simulink model "llr"  (R2020b)
settings: Solver=VariableStepAuto  StartTime=0.0  StopTime=20  RelTol=1e-3
values from neighbouring files (symbols this model uses):
  fs = 160e6    (= 160000000)    [setup.m]
libraries: simulink x14, hdlsllib x6, dspsigops x4, dspsrcs4 x3
settings Model: Creator=ckb13136  LastModifiedBy=ckb13136

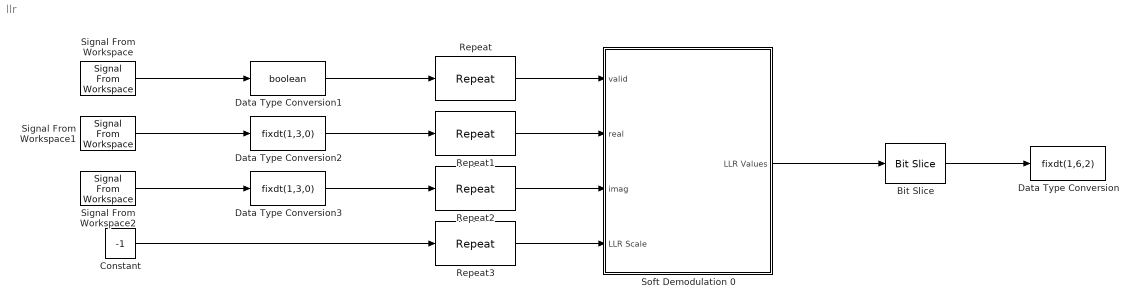
== system llr ==
  Bit Slice : hdlsllib/Logic and Bit Operations/Bit Slice  lidx=5  ridx=0
      settings: SourceProductBaseCode=SL
  Constant : Constant  Value=-1  OutDataTypeStr=fixdt(1,32,22)  SampleTime=1
  Data Type Conversion : DataTypeConversion  OutDataTypeStr=fixdt(1,6,2)  ConvertRealWorld=Stored Integer (SI)
  Data Type Conversion1 : DataTypeConversion  OutDataTypeStr=boolean
  Data Type Conversion2 : DataTypeConversion  OutDataTypeStr=fixdt(1,3,0)
  Data Type Conversion3 : DataTypeConversion  OutDataTypeStr=fixdt(1,3,0)
  Repeat{,1..3} (4 alike) : dspsigops/Repeat  N=4  InputProcessing=Columns as channels (frame based)  RateOptions=Allow multirate processing  ic=0  mode=Unused parameter value
      settings: SourceProductName=DSP System Toolbox
  Signal From Workspace : dspsrcs4/Signal From Workspace  X=ones(1,16)  Ts=1  nsamps=1  OutputAfterFinalValue=Setting to zero  ignoreOrWarnInputAndFrameLengths=off  OutputFrames=off
  Signal From Workspace1 : dspsrcs4/Signal From Workspace  X=[3 1 -1 -3 3 1 -1 -3 3 1 -1 -3 3 1 -1 -3 3 1 -1 -3 3 1 -1 -3]  Ts=1  nsamps=1  OutputAfterFinalValue=Setting to zero  ignoreOrWarnInputAndFrameLengths=off  OutputFrames=off
  Signal From Workspace2 : dspsrcs4/Signal From Workspace  X=[1 1 1 1 3 3 3 3 -1 -1 -1 -1 -3 -3 -3 -3]  Ts=1  nsamps=1  OutputAfterFinalValue=Setting to zero  ignoreOrWarnInputAndFrameLengths=off  OutputFrames=off
  Soft Demodulation 0 : Subsystem  mask{w=3, f=0, n=1}
  wires:
  Constant/1 -> Repeat3/1
  Signal From Workspace2/1 -> Data Type Conversion3/1
  Signal From Workspace1/1 -> Data Type Conversion2/1
  Signal From Workspace/1 -> Data Type Conversion1/1
  Soft Demodulation 0/1(LLR Values) -> Bit Slice/1
  Bit Slice/1 -> Data Type Conversion/1
  Repeat/1 -> Soft Demodulation 0/1(valid)
  Repeat1/1 -> Soft Demodulation 0/2(real)
  Repeat2/1 -> Soft Demodulation 0/3(imag)
  Repeat3/1 -> Soft Demodulation 0/4(LLR Scale)
  Data Type Conversion1/1 -> Repeat/1
  Data Type Conversion2/1 -> Repeat1/1
  Data Type Conversion3/1 -> Repeat2/1

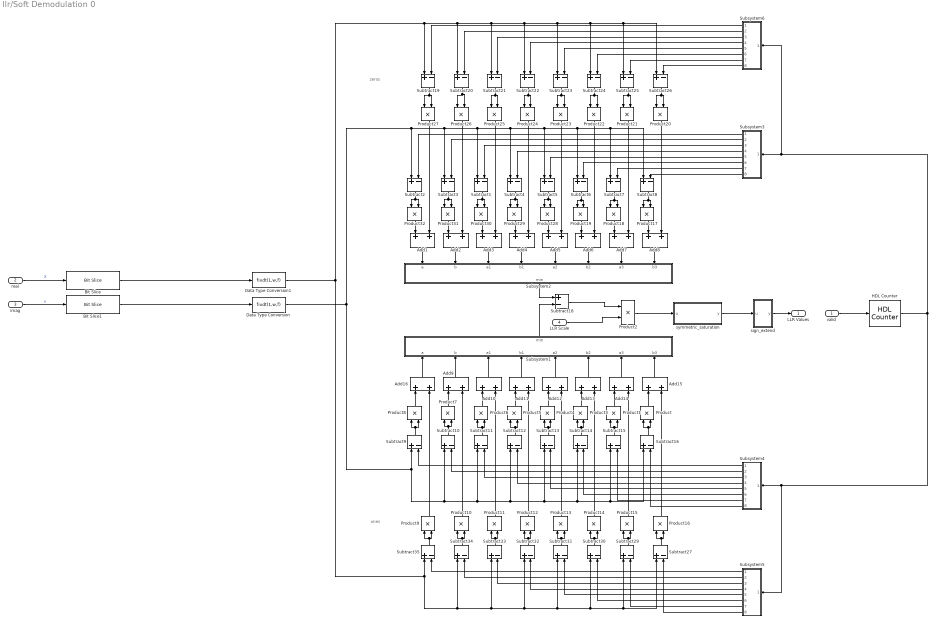
== system llr/Soft Demodulation 0 ==
  note: zeros
  note: ones
  valid : Inport
  real : Inport  Port=2
  imag : Inport  Port=3
  LLR Scale : Inport  Port=4
  Add{1..16} (16 alike) : Sum  OutDataTypeStr=fixdt(1,(w+1)*2+1,f*2)  SaturateOnIntegerOverflow=on
  Bit Slice : hdlsllib/Logic and Bit Operations/Bit Slice  lidx=(n*w)-1  ridx=(n-1)*w
      settings: SourceProductBaseCode=SL
  Bit Slice1 : hdlsllib/Logic and Bit Operations/Bit Slice  lidx=(n*w)-1  ridx=(n-1)*w
      settings: SourceProductBaseCode=SL
  Data Type Conversion : DataTypeConversion  OutDataTypeStr=fixdt(1,w,f)  ConvertRealWorld=Stored Integer (SI)
  Data Type Conversion1 : DataTypeConversion  OutDataTypeStr=fixdt(1,w,f)  ConvertRealWorld=Stored Integer (SI)
  HDL Counter : hdlsllib/Sources/HDL Counter  CountType=Count limited  CountInit=0  CountStep=1  CountMax=3  CountFromType=Initial value  CountFrom=0  CountResetPort=off  CountLoadPort=off  CountEnbPort=on  CountDirPort=off  CountDataType=Unsigned  CountWordLen=2  CountFracLen=0  CountSampTime=1/(fs*2)
  Product{,1,3..16} (16 alike) : Product  SaturateOnIntegerOverflow=on
  Product{17..32} (16 alike) : Product
  Product2 : Product  RndMeth=Round  SaturateOnIntegerOverflow=on
  Subsystem1 : Subsystem
  Subsystem2 : Subsystem
  Subsystem3 : Subsystem
  Subsystem4 : Subsystem
  Subsystem5 : Subsystem
  Subsystem6 : Subsystem
  Subtract{1..16,19..27,29..35} (32 alike) : Sum  Inputs=+-  OutDataTypeStr=fixdt(1,w+1,f)  SaturateOnIntegerOverflow=on
  Subtract18 : Sum  Inputs=+-  OutDataTypeStr=fixdt(1,(w+1)*2+2,f*2)  SaturateOnIntegerOverflow=on
  sign_extend : Subsystem
  symmetric_saturation : MATLAB Function  TreatAsAtomicUnit=on
  LLR Values : Outport
  wires:
  Subsystem5/4(Out4) -> Subtract32/2
  Product6/1 -> Add10/1
  Product10/1 -> Add9/2
  Add12/1 -> Subsystem1/5(a2)
  Product1/1 -> Add14/1
  Subtract13/1 -> Product4/1, Product4/2
  Product/1 -> Add15/1
  Add1/1 -> Subsystem2/1(a)
  Product20/1 -> Add8/2
  Add3/1 -> Subsystem2/3(a1)
  Subsystem2/1(min) -> Subtract18/1
  Subsystem3/6(Out6) -> Subtract6/2
  Subtract10/1 -> Product7/2, Product7/1
  Subtract35/1 -> Product9/2, Product9/1
  real/1 -> Bit Slice/1  "X"
  Product25/1 -> Add3/2
  Product19/1 -> Add6/1
  Product3/1 -> Add13/1
  Add7/1 -> Subsystem2/7(a3)
  Product23/1 -> Add5/2
  Subtract21/1 -> Product25/1, Product25/2
  Product4/1 -> Add12/1
  LLR Scale/1 -> Product2/2
  Add10/1 -> Subsystem1/3(a1)
  Subtract24/1 -> Product22/1, Product22/2
  Subtract1/1 -> Product30/1, Product30/2
  Subsystem4/6(Out6) -> Subtract14/2
  Subtract18/1 -> Product2/1
  Product5/1 -> Add11/1
  Subsystem1/1(min) -> Subtract18/2
  Product22/1 -> Add6/2
  Subsystem3/2(Out2) -> Subtract3/2
  Add13/1 -> Subsystem1/6(b2)
  Product26/1 -> Add2/2
  Subtract19/1 -> Product27/1, Product27/2
  Product31/1 -> Add2/1
  Subsystem3/5(Out5) -> Subtract5/2
  Product30/1 -> Add3/1
  Add15/1 -> Subsystem1/8(b3)
  Product18/1 -> Add7/1
  Subtract4/1 -> Product29/2, Product29/1
  Subtract5/1 -> Product28/1, Product28/2
  Subtract2/1 -> Product32/1, Product32/2
  Add16/1 -> Subsystem1/1(a)
  imag/1 -> Bit Slice1/1  "y"
  Add14/1 -> Subsystem1/7(a3)
  Subtract23/1 -> Product23/2, Product23/1
  Subtract15/1 -> Product1/2, Product1/1
  Subtract9/1 -> Product8/2, Product8/1
  Subsystem3/1(Out1) -> Subtract2/2
  Product27/1 -> Add1/2
  Add8/1 -> Subsystem2/8(b3)
  Product14/1 -> Add13/2
  Product15/1 -> Add14/2
  Add2/1 -> Subsystem2/2(b)
  Add11/1 -> Subsystem1/4(b1)
  Add6/1 -> Subsystem2/6(b2)
  Subtract25/1 -> Product21/1, Product21/2
  Product21/1 -> Add7/2
  Subsystem3/4(Out4) -> Subtract4/2
  Subsystem4/5(Out5) -> Subtract13/2
  Product7/1 -> Add9/1
  Product8/1 -> Add16/1
  Product12/1 -> Add11/2
  Product28/1 -> Add5/1
  Subsystem3/3(Out3) -> Subtract1/2
  Subtract26/1 -> Product20/1, Product20/2
  Subsystem4/7(Out7) -> Subtract15/2
  Add9/1 -> Subsystem1/2(b)
  Product9/1 -> Add16/2
  Subsystem4/4(Out4) -> Subtract12/2
  Product17/1 -> Add8/1
  Subsystem4/3(Out3) -> Subtract11/2
  Subsystem5/2(Out2) -> Subtract34/2
  Subsystem5/3(Out3) -> Subtract33/2
  Product13/1 -> Add12/2
  Subtract3/1 -> Product31/1, Product31/2
  Product24/1 -> Add4/2
  Subsystem5/6(Out6) -> Subtract30/2
  Subsystem4/1(Out1) -> Subtract9/2
  Product16/1 -> Add15/2
  Subsystem3/7(Out7) -> Subtract7/2
  Subtract12/1 -> Product5/2, Product5/1
  Subsystem5/1(Out1) -> Subtract35/2
  Product32/1 -> Add1/1
  Subtract34/1 -> Product10/2, Product10/1
  Subtract11/1 -> Product6/2, Product6/1
  Subsystem5/7(Out7) -> Subtract29/2
  Subsystem5/8(Out8) -> Subtract27/2
  Subsystem4/2(Out2) -> Subtract10/2
  Subsystem4/8(Out8) -> Subtract16/2
  Product29/1 -> Add4/1
  Product11/1 -> Add10/2
  Add4/1 -> Subsystem2/4(b1)
  Subsystem3/8(Out8) -> Subtract8/2
  Add5/1 -> Subsystem2/5(a2)
  Subtract16/1 -> Product/2, Product/1
  Subsystem5/5(Out5) -> Subtract31/2
  Subtract14/1 -> Product3/1, Product3/2
  Subtract33/1 -> Product11/1, Product11/2
  Subtract32/1 -> Product12/1, Product12/2
  Subtract31/1 -> Product13/1, Product13/2
  Subtract30/1 -> Product14/1, Product14/2
  Subtract29/1 -> Product15/1, Product15/2
  Subtract27/1 -> Product16/1, Product16/2
  Subtract8/1 -> Product17/2, Product17/1
  Subtract7/1 -> Product18/1, Product18/2
  Subtract20/1 -> Product26/2, Product26/1
  Subtract22/1 -> Product24/1, Product24/2
  Subtract6/1 -> Product19/1, Product19/2
  Subsystem6/1(Out1) -> Subtract19/2
  Subsystem6/2(Out2) -> Subtract20/2
  Subsystem6/3(Out3) -> Subtract21/2
  Subsystem6/4(Out4) -> Subtract22/2
  Subsystem6/5(Out5) -> Subtract23/2
  Subsystem6/6(Out6) -> Subtract24/2
  Subsystem6/7(Out7) -> Subtract25/2
  Subsystem6/8(Out8) -> Subtract26/2
  valid/1 -> HDL Counter/1
  HDL Counter/1 -> Subsystem5/1(enb), Subsystem4/1(enb), Subsystem6/1(enb), Subsystem3/1(enb)
  symmetric_saturation/1(y) -> sign_extend/1(u)
  Product2/1 -> symmetric_saturation/1(u)
  sign_extend/1(y) -> LLR Values/1
  Data Type Conversion/1 -> Subtract2/1, Subtract3/1, Subtract1/1, Subtract4/1, Subtract5/1, Subtract6/1, Subtract8/1, Subtract7/1, Subtract9/1, Subtract10/1, Subtract11/1, Subtract12/1, Subtract13/1, Subtract14/1, Subtract16/1, Subtract15/1
  Data Type Conversion1/1 -> Subtract19/1, Subtract21/1, Subtract22/1, Subtract23/1, Subtract24/1, Subtract25/1, Subtract26/1, Subtract20/1, Subtract35/1, Subtract34/1, Subtract33/1, Subtract32/1, Subtract31/1, Subtract30/1, Subtract29/1, Subtract27/1
  Bit Slice1/1 -> Data Type Conversion/1
  Bit Slice/1 -> Data Type Conversion1/1

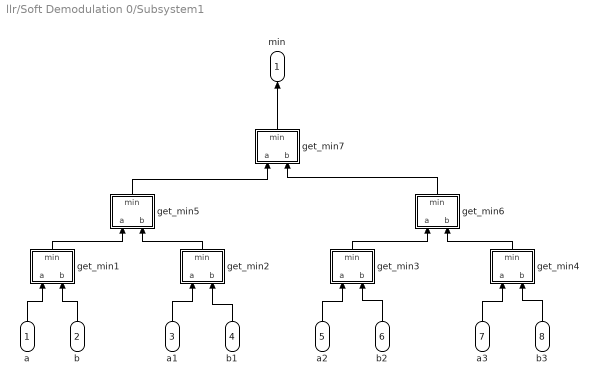
== system llr/Soft Demodulation 0/Subsystem1 ==
  a : Inport
  b : Inport  Port=2
  a1 : Inport  Port=3
  b1 : Inport  Port=4
  a2 : Inport  Port=5
  b2 : Inport  Port=6
  a3 : Inport  Port=7
  b3 : Inport  Port=8
  get_min1 : Subsystem
  get_min2 : Subsystem
  get_min3 : Subsystem
  get_min4 : Subsystem
  get_min5 : Subsystem
  get_min6 : Subsystem
  get_min7 : Subsystem
  min : Outport
  wires:
  get_min5/1(min) -> get_min7/1(a)
  b2/1 -> get_min3/2(b)
  a/1 -> get_min1/1(a)
  get_min6/1(min) -> get_min7/2(b)
  get_min3/1(min) -> get_min6/1(a)
  b1/1 -> get_min2/2(b)
  get_min2/1(min) -> get_min5/2(b)
  get_min4/1(min) -> get_min6/2(b)
  a3/1 -> get_min4/1(a)
  get_min1/1(min) -> get_min5/1(a)
  get_min7/1(min) -> min/1
  b3/1 -> get_min4/2(b)
  a1/1 -> get_min2/1(a)
  b/1 -> get_min1/2(b)
  a2/1 -> get_min3/1(a)

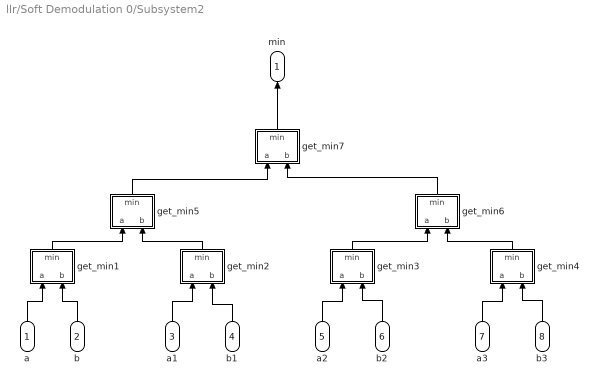
== system llr/Soft Demodulation 0/Subsystem2 ==
  a : Inport
  b : Inport  Port=2
  a1 : Inport  Port=3
  b1 : Inport  Port=4
  a2 : Inport  Port=5
  b2 : Inport  Port=6
  a3 : Inport  Port=7
  b3 : Inport  Port=8
  get_min1 : Subsystem
  get_min2 : Subsystem
  get_min3 : Subsystem
  get_min4 : Subsystem
  get_min5 : Subsystem
  get_min6 : Subsystem
  get_min7 : Subsystem
  min : Outport
  wires:
  get_min5/1(min) -> get_min7/1(a)
  b2/1 -> get_min3/2(b)
  a/1 -> get_min1/1(a)
  get_min6/1(min) -> get_min7/2(b)
  get_min3/1(min) -> get_min6/1(a)
  b1/1 -> get_min2/2(b)
  get_min2/1(min) -> get_min5/2(b)
  get_min4/1(min) -> get_min6/2(b)
  a3/1 -> get_min4/1(a)
  get_min1/1(min) -> get_min5/1(a)
  get_min7/1(min) -> min/1
  b3/1 -> get_min4/2(b)
  a1/1 -> get_min2/1(a)
  b/1 -> get_min1/2(b)
  a2/1 -> get_min3/1(a)

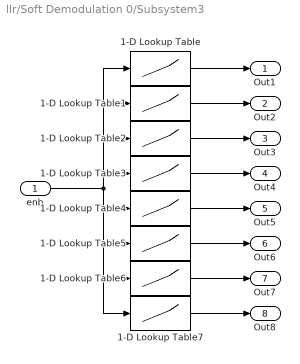
== system llr/Soft Demodulation 0/Subsystem3 ==
  enb : Inport
  1-D Lookup Table : Lookup_n-D  NumberOfTableDimensions=1  BreakpointsForDimension1=[0:3]  IndexSearchMethod=Evenly spaced points  Table=z_y(1:8:end)  InterpMethod=Flat  DiagnosticForOutOfRangeInput=Error  InternalRulePriority=Speed  OutDataTypeStr=fixdt(1,3,0)  RndMeth=Simplest  InputSameDT=on
  1-D Lookup Table1 : Lookup_n-D  NumberOfTableDimensions=1  BreakpointsForDimension1=[0:3]  IndexSearchMethod=Evenly spaced points  Table=z_y(2:8:end)  InterpMethod=Flat  DiagnosticForOutOfRangeInput=Error  InternalRulePriority=Speed  OutDataTypeStr=fixdt(1,3,0)  RndMeth=Simplest  InputSameDT=on
  1-D Lookup Table2 : Lookup_n-D  NumberOfTableDimensions=1  BreakpointsForDimension1=[0:3]  IndexSearchMethod=Evenly spaced points  Table=z_y(3:8:end)  InterpMethod=Flat  DiagnosticForOutOfRangeInput=Error  InternalRulePriority=Speed  OutDataTypeStr=fixdt(1,3,0)  RndMeth=Simplest  InputSameDT=on
  1-D Lookup Table3 : Lookup_n-D  NumberOfTableDimensions=1  BreakpointsForDimension1=[0:3]  IndexSearchMethod=Evenly spaced points  Table=z_y(4:8:end)  InterpMethod=Flat  DiagnosticForOutOfRangeInput=Error  InternalRulePriority=Speed  OutDataTypeStr=fixdt(1,3,0)  RndMeth=Simplest  InputSameDT=on
  1-D Lookup Table4 : Lookup_n-D  NumberOfTableDimensions=1  BreakpointsForDimension1=[0:3]  IndexSearchMethod=Evenly spaced points  Table=z_y(5:8:end)  InterpMethod=Flat  DiagnosticForOutOfRangeInput=Error  InternalRulePriority=Speed  OutDataTypeStr=fixdt(1,3,0)  RndMeth=Simplest  InputSameDT=on
  1-D Lookup Table5 : Lookup_n-D  NumberOfTableDimensions=1  BreakpointsForDimension1=[0:3]  IndexSearchMethod=Evenly spaced points  Table=z_y(6:8:end)  InterpMethod=Flat  DiagnosticForOutOfRangeInput=Error  InternalRulePriority=Speed  OutDataTypeStr=fixdt(1,3,0)  RndMeth=Simplest  InputSameDT=on
  1-D Lookup Table6 : Lookup_n-D  NumberOfTableDimensions=1  BreakpointsForDimension1=[0:3]  IndexSearchMethod=Evenly spaced points  Table=z_y(7:8:end)  InterpMethod=Flat  DiagnosticForOutOfRangeInput=Error  InternalRulePriority=Speed  OutDataTypeStr=fixdt(1,3,0)  RndMeth=Simplest  InputSameDT=on
  1-D Lookup Table7 : Lookup_n-D  NumberOfTableDimensions=1  BreakpointsForDimension1=[0:3]  IndexSearchMethod=Evenly spaced points  Table=z_y(8:8:end)  InterpMethod=Flat  DiagnosticForOutOfRangeInput=Error  InternalRulePriority=Speed  OutDataTypeStr=fixdt(1,3,0)  RndMeth=Simplest  InputSameDT=on
  Out1 : Outport
  Out2 : Outport  Port=2
  Out3 : Outport  Port=3
  Out4 : Outport  Port=4
  Out5 : Outport  Port=5
  Out6 : Outport  Port=6
  Out7 : Outport  Port=7
  Out8 : Outport  Port=8
  wires:
  1-D Lookup Table6/1 -> Out7/1
  enb/1 -> 1-D Lookup Table4/1, 1-D Lookup Table5/1, 1-D Lookup Table6/1, 1-D Lookup Table7/1, 1-D Lookup Table/1, 1-D Lookup Table1/1, 1-D Lookup Table2/1, 1-D Lookup Table3/1
  1-D Lookup Table3/1 -> Out4/1
  1-D Lookup Table1/1 -> Out2/1
  1-D Lookup Table4/1 -> Out5/1
  1-D Lookup Table5/1 -> Out6/1
  1-D Lookup Table/1 -> Out1/1
  1-D Lookup Table2/1 -> Out3/1
  1-D Lookup Table7/1 -> Out8/1

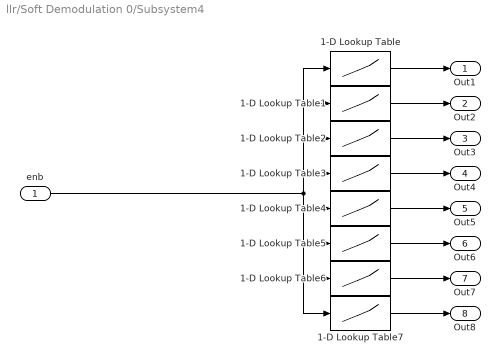
== system llr/Soft Demodulation 0/Subsystem4 ==
  enb : Inport
  1-D Lookup Table : Lookup_n-D  NumberOfTableDimensions=1  BreakpointsForDimension1=[0:3]  IndexSearchMethod=Evenly spaced points  Table=o_y(1:8:end)  InterpMethod=Flat  DiagnosticForOutOfRangeInput=Error  InternalRulePriority=Speed  OutDataTypeStr=fixdt(1,3,0)  RndMeth=Simplest  InputSameDT=on
  1-D Lookup Table1 : Lookup_n-D  NumberOfTableDimensions=1  BreakpointsForDimension1=[0:3]  IndexSearchMethod=Evenly spaced points  Table=o_y(2:8:end)  InterpMethod=Flat  DiagnosticForOutOfRangeInput=Error  InternalRulePriority=Speed  OutDataTypeStr=fixdt(1,3,0)  RndMeth=Simplest  InputSameDT=on
  1-D Lookup Table2 : Lookup_n-D  NumberOfTableDimensions=1  BreakpointsForDimension1=[0:3]  IndexSearchMethod=Evenly spaced points  Table=o_y(3:8:end)  InterpMethod=Flat  DiagnosticForOutOfRangeInput=Error  InternalRulePriority=Speed  OutDataTypeStr=fixdt(1,3,0)  RndMeth=Simplest  InputSameDT=on
  1-D Lookup Table3 : Lookup_n-D  NumberOfTableDimensions=1  BreakpointsForDimension1=[0:3]  IndexSearchMethod=Evenly spaced points  Table=o_y(4:8:end)  InterpMethod=Flat  DiagnosticForOutOfRangeInput=Error  InternalRulePriority=Speed  OutDataTypeStr=fixdt(1,3,0)  RndMeth=Simplest  InputSameDT=on
  1-D Lookup Table4 : Lookup_n-D  NumberOfTableDimensions=1  BreakpointsForDimension1=[0:3]  IndexSearchMethod=Evenly spaced points  Table=o_y(5:8:end)  InterpMethod=Flat  DiagnosticForOutOfRangeInput=Error  InternalRulePriority=Speed  OutDataTypeStr=fixdt(1,3,0)  RndMeth=Simplest  InputSameDT=on
  1-D Lookup Table5 : Lookup_n-D  NumberOfTableDimensions=1  BreakpointsForDimension1=[0:3]  IndexSearchMethod=Evenly spaced points  Table=o_y(6:8:end)  InterpMethod=Flat  DiagnosticForOutOfRangeInput=Error  InternalRulePriority=Speed  OutDataTypeStr=fixdt(1,3,0)  RndMeth=Simplest  InputSameDT=on
  1-D Lookup Table6 : Lookup_n-D  NumberOfTableDimensions=1  BreakpointsForDimension1=[0:3]  IndexSearchMethod=Evenly spaced points  Table=o_y(7:8:end)  InterpMethod=Flat  DiagnosticForOutOfRangeInput=Error  InternalRulePriority=Speed  OutDataTypeStr=fixdt(1,3,0)  RndMeth=Simplest  InputSameDT=on
  1-D Lookup Table7 : Lookup_n-D  NumberOfTableDimensions=1  BreakpointsForDimension1=[0:3]  IndexSearchMethod=Evenly spaced points  Table=o_y(8:8:end)  InterpMethod=Flat  DiagnosticForOutOfRangeInput=Error  InternalRulePriority=Speed  OutDataTypeStr=fixdt(1,3,0)  RndMeth=Simplest  InputSameDT=on
  Out1 : Outport
  Out2 : Outport  Port=2
  Out3 : Outport  Port=3
  Out4 : Outport  Port=4
  Out5 : Outport  Port=5
  Out6 : Outport  Port=6
  Out7 : Outport  Port=7
  Out8 : Outport  Port=8
  wires:
  1-D Lookup Table7/1 -> Out8/1
  1-D Lookup Table2/1 -> Out3/1
  1-D Lookup Table/1 -> Out1/1
  1-D Lookup Table5/1 -> Out6/1
  1-D Lookup Table4/1 -> Out5/1
  1-D Lookup Table1/1 -> Out2/1
  1-D Lookup Table3/1 -> Out4/1
  enb/1 -> 1-D Lookup Table7/1, 1-D Lookup Table6/1, 1-D Lookup Table5/1, 1-D Lookup Table4/1, 1-D Lookup Table3/1, 1-D Lookup Table2/1, 1-D Lookup Table1/1, 1-D Lookup Table/1
  1-D Lookup Table6/1 -> Out7/1

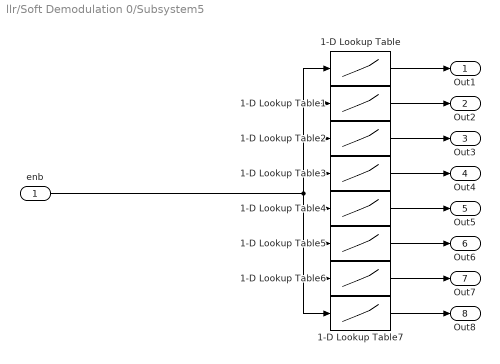
== system llr/Soft Demodulation 0/Subsystem5 ==
  enb : Inport
  1-D Lookup Table : Lookup_n-D  NumberOfTableDimensions=1  BreakpointsForDimension1=[0:3]  IndexSearchMethod=Evenly spaced points  Table=o_x(1:8:end)  InterpMethod=Flat  DiagnosticForOutOfRangeInput=Error  InternalRulePriority=Speed  OutDataTypeStr=fixdt(1,3,0)  RndMeth=Simplest  InputSameDT=on
  1-D Lookup Table1 : Lookup_n-D  NumberOfTableDimensions=1  BreakpointsForDimension1=[0:3]  IndexSearchMethod=Evenly spaced points  Table=o_x(2:8:end)  InterpMethod=Flat  DiagnosticForOutOfRangeInput=Error  InternalRulePriority=Speed  OutDataTypeStr=fixdt(1,3,0)  RndMeth=Simplest  InputSameDT=on
  1-D Lookup Table2 : Lookup_n-D  NumberOfTableDimensions=1  BreakpointsForDimension1=[0:3]  IndexSearchMethod=Evenly spaced points  Table=o_x(3:8:end)  InterpMethod=Flat  DiagnosticForOutOfRangeInput=Error  InternalRulePriority=Speed  OutDataTypeStr=fixdt(1,3,0)  RndMeth=Simplest  InputSameDT=on
  1-D Lookup Table3 : Lookup_n-D  NumberOfTableDimensions=1  BreakpointsForDimension1=[0:3]  IndexSearchMethod=Evenly spaced points  Table=o_x(4:8:end)  InterpMethod=Flat  DiagnosticForOutOfRangeInput=Error  InternalRulePriority=Speed  OutDataTypeStr=fixdt(1,3,0)  RndMeth=Simplest  InputSameDT=on
  1-D Lookup Table4 : Lookup_n-D  NumberOfTableDimensions=1  BreakpointsForDimension1=[0:3]  IndexSearchMethod=Evenly spaced points  Table=o_x(5:8:end)  InterpMethod=Flat  DiagnosticForOutOfRangeInput=Error  InternalRulePriority=Speed  OutDataTypeStr=fixdt(1,3,0)  RndMeth=Simplest  InputSameDT=on
  1-D Lookup Table5 : Lookup_n-D  NumberOfTableDimensions=1  BreakpointsForDimension1=[0:3]  IndexSearchMethod=Evenly spaced points  Table=o_x(6:8:end)  InterpMethod=Flat  DiagnosticForOutOfRangeInput=Error  InternalRulePriority=Speed  OutDataTypeStr=fixdt(1,3,0)  RndMeth=Simplest  InputSameDT=on
  1-D Lookup Table6 : Lookup_n-D  NumberOfTableDimensions=1  BreakpointsForDimension1=[0:3]  IndexSearchMethod=Evenly spaced points  Table=o_x(7:8:end)  InterpMethod=Flat  DiagnosticForOutOfRangeInput=Error  InternalRulePriority=Speed  OutDataTypeStr=fixdt(1,3,0)  RndMeth=Simplest  InputSameDT=on
  1-D Lookup Table7 : Lookup_n-D  NumberOfTableDimensions=1  BreakpointsForDimension1=[0:3]  IndexSearchMethod=Evenly spaced points  Table=o_x(8:8:end)  InterpMethod=Flat  DiagnosticForOutOfRangeInput=Error  InternalRulePriority=Speed  OutDataTypeStr=fixdt(1,3,0)  RndMeth=Simplest  InputSameDT=on
  Out1 : Outport
  Out2 : Outport  Port=2
  Out3 : Outport  Port=3
  Out4 : Outport  Port=4
  Out5 : Outport  Port=5
  Out6 : Outport  Port=6
  Out7 : Outport  Port=7
  Out8 : Outport  Port=8
  wires:
  1-D Lookup Table6/1 -> Out7/1
  enb/1 -> 1-D Lookup Table/1, 1-D Lookup Table1/1, 1-D Lookup Table2/1, 1-D Lookup Table3/1, 1-D Lookup Table4/1, 1-D Lookup Table5/1, 1-D Lookup Table6/1, 1-D Lookup Table7/1
  1-D Lookup Table3/1 -> Out4/1
  1-D Lookup Table1/1 -> Out2/1
  1-D Lookup Table4/1 -> Out5/1
  1-D Lookup Table5/1 -> Out6/1
  1-D Lookup Table/1 -> Out1/1
  1-D Lookup Table2/1 -> Out3/1
  1-D Lookup Table7/1 -> Out8/1

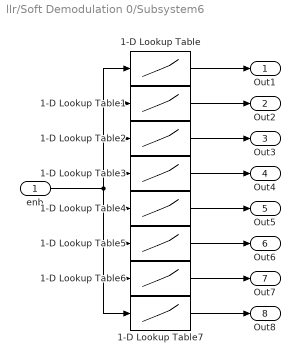
== system llr/Soft Demodulation 0/Subsystem6 ==
  enb : Inport
  1-D Lookup Table : Lookup_n-D  NumberOfTableDimensions=1  BreakpointsForDimension1=[0:3]  IndexSearchMethod=Evenly spaced points  Table=z_x(1:8:end)  InterpMethod=Flat  DiagnosticForOutOfRangeInput=Error  InternalRulePriority=Speed  OutDataTypeStr=fixdt(1,3,0)  RndMeth=Simplest  InputSameDT=on
  1-D Lookup Table1 : Lookup_n-D  NumberOfTableDimensions=1  BreakpointsForDimension1=[0:3]  IndexSearchMethod=Evenly spaced points  Table=z_x(2:8:end)  InterpMethod=Flat  DiagnosticForOutOfRangeInput=Error  InternalRulePriority=Speed  OutDataTypeStr=fixdt(1,3,0)  RndMeth=Simplest  InputSameDT=on
  1-D Lookup Table2 : Lookup_n-D  NumberOfTableDimensions=1  BreakpointsForDimension1=[0:3]  IndexSearchMethod=Evenly spaced points  Table=z_x(3:8:end)  InterpMethod=Flat  DiagnosticForOutOfRangeInput=Error  InternalRulePriority=Speed  OutDataTypeStr=fixdt(1,3,0)  RndMeth=Simplest  InputSameDT=on
  1-D Lookup Table3 : Lookup_n-D  NumberOfTableDimensions=1  BreakpointsForDimension1=[0:3]  IndexSearchMethod=Evenly spaced points  Table=z_x(4:8:end)  InterpMethod=Flat  DiagnosticForOutOfRangeInput=Error  InternalRulePriority=Speed  OutDataTypeStr=fixdt(1,3,0)  RndMeth=Simplest  InputSameDT=on
  1-D Lookup Table4 : Lookup_n-D  NumberOfTableDimensions=1  BreakpointsForDimension1=[0:3]  IndexSearchMethod=Evenly spaced points  Table=z_x(5:8:end)  InterpMethod=Flat  DiagnosticForOutOfRangeInput=Error  InternalRulePriority=Speed  OutDataTypeStr=fixdt(1,3,0)  RndMeth=Simplest  InputSameDT=on
  1-D Lookup Table5 : Lookup_n-D  NumberOfTableDimensions=1  BreakpointsForDimension1=[0:3]  IndexSearchMethod=Evenly spaced points  Table=z_x(6:8:end)  InterpMethod=Flat  DiagnosticForOutOfRangeInput=Error  InternalRulePriority=Speed  OutDataTypeStr=fixdt(1,3,0)  RndMeth=Simplest  InputSameDT=on
  1-D Lookup Table6 : Lookup_n-D  NumberOfTableDimensions=1  BreakpointsForDimension1=[0:3]  IndexSearchMethod=Evenly spaced points  Table=z_x(7:8:end)  InterpMethod=Flat  DiagnosticForOutOfRangeInput=Error  InternalRulePriority=Speed  OutDataTypeStr=fixdt(1,3,0)  RndMeth=Simplest  InputSameDT=on
  1-D Lookup Table7 : Lookup_n-D  NumberOfTableDimensions=1  BreakpointsForDimension1=[0:3]  IndexSearchMethod=Evenly spaced points  Table=z_x(8:8:end)  InterpMethod=Flat  DiagnosticForOutOfRangeInput=Error  InternalRulePriority=Speed  OutDataTypeStr=fixdt(1,3,0)  RndMeth=Simplest  InputSameDT=on
  Out1 : Outport
  Out2 : Outport  Port=2
  Out3 : Outport  Port=3
  Out4 : Outport  Port=4
  Out5 : Outport  Port=5
  Out6 : Outport  Port=6
  Out7 : Outport  Port=7
  Out8 : Outport  Port=8
  wires:
  1-D Lookup Table7/1 -> Out8/1
  1-D Lookup Table2/1 -> Out3/1
  1-D Lookup Table/1 -> Out1/1
  1-D Lookup Table5/1 -> Out6/1
  1-D Lookup Table4/1 -> Out5/1
  1-D Lookup Table1/1 -> Out2/1
  1-D Lookup Table3/1 -> Out4/1
  enb/1 -> 1-D Lookup Table3/1, 1-D Lookup Table2/1, 1-D Lookup Table1/1, 1-D Lookup Table/1, 1-D Lookup Table7/1, 1-D Lookup Table6/1, 1-D Lookup Table5/1, 1-D Lookup Table4/1
  1-D Lookup Table6/1 -> Out7/1

== system llr/Soft Demodulation 0/sign_extend ==
  u : Inport
  Bit Concat : hdlsllib/Logic and Bit Operations/Bit Concat  numInputs=3
  Bit Slice : hdlsllib/Logic and Bit Operations/Bit Slice  lidx=5  ridx=5
      settings: SourceProductBaseCode=SL
  y : Outport
  wires:
  Bit Slice/1 -> Bit Concat/1, Bit Concat/2
  u/1 -> Bit Slice/1, Bit Concat/3
  Bit Concat/1 -> y/1

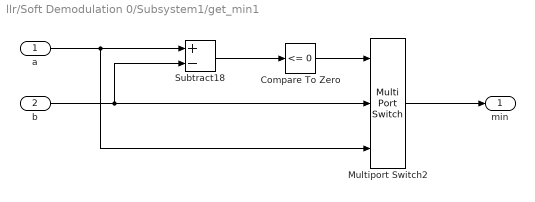
== system llr/Soft Demodulation 0/Subsystem1/get_min1 ==
  a : Inport
  b : Inport  Port=2
  Compare To Zero : simulink/Logic and Bit Operations/Compare To Zero  relop=<=  OutDataTypeStr=boolean
  Multiport Switch2 : MultiPortSwitch  DataPortOrder=Zero-based contiguous  Inputs=2  zeroidx=on
  Subtract18 : Sum  Inputs=+-  OutDataTypeStr=fixdt(1,(w+1)*2+2,f*2)  SaturateOnIntegerOverflow=on
  min : Outport
  wires:
  Subtract18/1 -> Compare To Zero/1
  b/1 -> Subtract18/2, Multiport Switch2/2
  a/1 -> Multiport Switch2/3, Subtract18/1
  Multiport Switch2/1 -> min/1
  Compare To Zero/1 -> Multiport Switch2/1

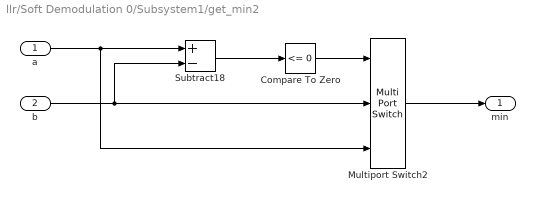
== system llr/Soft Demodulation 0/Subsystem1/get_min2 ==
  a : Inport
  b : Inport  Port=2
  Compare To Zero : simulink/Logic and Bit Operations/Compare To Zero  relop=<=  OutDataTypeStr=boolean
  Multiport Switch2 : MultiPortSwitch  DataPortOrder=Zero-based contiguous  Inputs=2  zeroidx=on
  Subtract18 : Sum  Inputs=+-  OutDataTypeStr=fixdt(1,(w+1)*2+2,f*2)  SaturateOnIntegerOverflow=on
  min : Outport
  wires:
  Compare To Zero/1 -> Multiport Switch2/1
  Multiport Switch2/1 -> min/1
  a/1 -> Subtract18/1, Multiport Switch2/3
  b/1 -> Multiport Switch2/2, Subtract18/2
  Subtract18/1 -> Compare To Zero/1

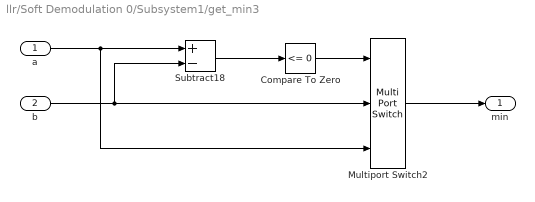
== system llr/Soft Demodulation 0/Subsystem1/get_min3 ==
  a : Inport
  b : Inport  Port=2
  Compare To Zero : simulink/Logic and Bit Operations/Compare To Zero  relop=<=  OutDataTypeStr=boolean
  Multiport Switch2 : MultiPortSwitch  DataPortOrder=Zero-based contiguous  Inputs=2  zeroidx=on
  Subtract18 : Sum  Inputs=+-  OutDataTypeStr=fixdt(1,(w+1)*2+2,f*2)  SaturateOnIntegerOverflow=on
  min : Outport
  wires:
  Subtract18/1 -> Compare To Zero/1
  b/1 -> Subtract18/2, Multiport Switch2/2
  a/1 -> Multiport Switch2/3, Subtract18/1
  Multiport Switch2/1 -> min/1
  Compare To Zero/1 -> Multiport Switch2/1

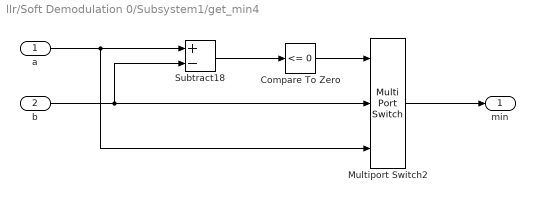
== system llr/Soft Demodulation 0/Subsystem1/get_min4 ==
  a : Inport
  b : Inport  Port=2
  Compare To Zero : simulink/Logic and Bit Operations/Compare To Zero  relop=<=  OutDataTypeStr=boolean
  Multiport Switch2 : MultiPortSwitch  DataPortOrder=Zero-based contiguous  Inputs=2  zeroidx=on
  Subtract18 : Sum  Inputs=+-  OutDataTypeStr=fixdt(1,(w+1)*2+2,f*2)  SaturateOnIntegerOverflow=on
  min : Outport
  wires:
  Compare To Zero/1 -> Multiport Switch2/1
  Multiport Switch2/1 -> min/1
  a/1 -> Subtract18/1, Multiport Switch2/3
  b/1 -> Multiport Switch2/2, Subtract18/2
  Subtract18/1 -> Compare To Zero/1

== system llr/Soft Demodulation 0/Subsystem1/get_min5 ==
  a : Inport
  b : Inport  Port=2
  Compare To Zero : simulink/Logic and Bit Operations/Compare To Zero  relop=<=  OutDataTypeStr=boolean
  Multiport Switch2 : MultiPortSwitch  DataPortOrder=Zero-based contiguous  Inputs=2  zeroidx=on
  Subtract18 : Sum  Inputs=+-  OutDataTypeStr=fixdt(1,(w+1)*2+2,f*2)  SaturateOnIntegerOverflow=on
  min : Outport
  wires:
  Subtract18/1 -> Compare To Zero/1
  b/1 -> Subtract18/2, Multiport Switch2/2
  a/1 -> Multiport Switch2/3, Subtract18/1
  Multiport Switch2/1 -> min/1
  Compare To Zero/1 -> Multiport Switch2/1

== system llr/Soft Demodulation 0/Subsystem1/get_min6 ==
  a : Inport
  b : Inport  Port=2
  Compare To Zero : simulink/Logic and Bit Operations/Compare To Zero  relop=<=  OutDataTypeStr=boolean
  Multiport Switch2 : MultiPortSwitch  DataPortOrder=Zero-based contiguous  Inputs=2  zeroidx=on
  Subtract18 : Sum  Inputs=+-  OutDataTypeStr=fixdt(1,(w+1)*2+2,f*2)  SaturateOnIntegerOverflow=on
  min : Outport
  wires:
  Compare To Zero/1 -> Multiport Switch2/1
  Multiport Switch2/1 -> min/1
  a/1 -> Subtract18/1, Multiport Switch2/3
  b/1 -> Multiport Switch2/2, Subtract18/2
  Subtract18/1 -> Compare To Zero/1

== system llr/Soft Demodulation 0/Subsystem1/get_min7 ==
  a : Inport
  b : Inport  Port=2
  Compare To Zero : simulink/Logic and Bit Operations/Compare To Zero  relop=<=  OutDataTypeStr=boolean
  Multiport Switch2 : MultiPortSwitch  DataPortOrder=Zero-based contiguous  Inputs=2  zeroidx=on
  Subtract18 : Sum  Inputs=+-  OutDataTypeStr=fixdt(1,(w+1)*2+2,f*2)  SaturateOnIntegerOverflow=on
  min : Outport
  wires:
  Compare To Zero/1 -> Multiport Switch2/1
  Multiport Switch2/1 -> min/1
  a/1 -> Subtract18/1, Multiport Switch2/3
  b/1 -> Multiport Switch2/2, Subtract18/2
  Subtract18/1 -> Compare To Zero/1

== system llr/Soft Demodulation 0/Subsystem2/get_min1 ==
  a : Inport
  b : Inport  Port=2
  Compare To Zero : simulink/Logic and Bit Operations/Compare To Zero  relop=<=  OutDataTypeStr=boolean
  Multiport Switch2 : MultiPortSwitch  DataPortOrder=Zero-based contiguous  Inputs=2  zeroidx=on
  Subtract18 : Sum  Inputs=+-  OutDataTypeStr=fixdt(1,(w+1)*2+2,f*2)  SaturateOnIntegerOverflow=on
  min : Outport
  wires:
  Subtract18/1 -> Compare To Zero/1
  b/1 -> Subtract18/2, Multiport Switch2/2
  a/1 -> Multiport Switch2/3, Subtract18/1
  Multiport Switch2/1 -> min/1
  Compare To Zero/1 -> Multiport Switch2/1

== system llr/Soft Demodulation 0/Subsystem2/get_min2 ==
  a : Inport
  b : Inport  Port=2
  Compare To Zero : simulink/Logic and Bit Operations/Compare To Zero  relop=<=  OutDataTypeStr=boolean
  Multiport Switch2 : MultiPortSwitch  DataPortOrder=Zero-based contiguous  Inputs=2  zeroidx=on
  Subtract18 : Sum  Inputs=+-  OutDataTypeStr=fixdt(1,(w+1)*2+2,f*2)  SaturateOnIntegerOverflow=on
  min : Outport
  wires:
  Compare To Zero/1 -> Multiport Switch2/1
  Multiport Switch2/1 -> min/1
  a/1 -> Subtract18/1, Multiport Switch2/3
  b/1 -> Multiport Switch2/2, Subtract18/2
  Subtract18/1 -> Compare To Zero/1

== system llr/Soft Demodulation 0/Subsystem2/get_min3 ==
  a : Inport
  b : Inport  Port=2
  Compare To Zero : simulink/Logic and Bit Operations/Compare To Zero  relop=<=  OutDataTypeStr=boolean
  Multiport Switch2 : MultiPortSwitch  DataPortOrder=Zero-based contiguous  Inputs=2  zeroidx=on
  Subtract18 : Sum  Inputs=+-  OutDataTypeStr=fixdt(1,(w+1)*2+2,f*2)  SaturateOnIntegerOverflow=on
  min : Outport
  wires:
  Subtract18/1 -> Compare To Zero/1
  b/1 -> Subtract18/2, Multiport Switch2/2
  a/1 -> Multiport Switch2/3, Subtract18/1
  Multiport Switch2/1 -> min/1
  Compare To Zero/1 -> Multiport Switch2/1

== system llr/Soft Demodulation 0/Subsystem2/get_min4 ==
  a : Inport
  b : Inport  Port=2
  Compare To Zero : simulink/Logic and Bit Operations/Compare To Zero  relop=<=  OutDataTypeStr=boolean
  Multiport Switch2 : MultiPortSwitch  DataPortOrder=Zero-based contiguous  Inputs=2  zeroidx=on
  Subtract18 : Sum  Inputs=+-  OutDataTypeStr=fixdt(1,(w+1)*2+2,f*2)  SaturateOnIntegerOverflow=on
  min : Outport
  wires:
  Compare To Zero/1 -> Multiport Switch2/1
  Multiport Switch2/1 -> min/1
  a/1 -> Subtract18/1, Multiport Switch2/3
  b/1 -> Multiport Switch2/2, Subtract18/2
  Subtract18/1 -> Compare To Zero/1

== system llr/Soft Demodulation 0/Subsystem2/get_min5 ==
  a : Inport
  b : Inport  Port=2
  Compare To Zero : simulink/Logic and Bit Operations/Compare To Zero  relop=<=  OutDataTypeStr=boolean
  Multiport Switch2 : MultiPortSwitch  DataPortOrder=Zero-based contiguous  Inputs=2  zeroidx=on
  Subtract18 : Sum  Inputs=+-  OutDataTypeStr=fixdt(1,(w+1)*2+2,f*2)  SaturateOnIntegerOverflow=on
  min : Outport
  wires:
  Subtract18/1 -> Compare To Zero/1
  b/1 -> Subtract18/2, Multiport Switch2/2
  a/1 -> Multiport Switch2/3, Subtract18/1
  Multiport Switch2/1 -> min/1
  Compare To Zero/1 -> Multiport Switch2/1

== system llr/Soft Demodulation 0/Subsystem2/get_min6 ==
  a : Inport
  b : Inport  Port=2
  Compare To Zero : simulink/Logic and Bit Operations/Compare To Zero  relop=<=  OutDataTypeStr=boolean
  Multiport Switch2 : MultiPortSwitch  DataPortOrder=Zero-based contiguous  Inputs=2  zeroidx=on
  Subtract18 : Sum  Inputs=+-  OutDataTypeStr=fixdt(1,(w+1)*2+2,f*2)  SaturateOnIntegerOverflow=on
  min : Outport
  wires:
  Compare To Zero/1 -> Multiport Switch2/1
  Multiport Switch2/1 -> min/1
  a/1 -> Subtract18/1, Multiport Switch2/3
  b/1 -> Multiport Switch2/2, Subtract18/2
  Subtract18/1 -> Compare To Zero/1

== system llr/Soft Demodulation 0/Subsystem2/get_min7 ==
  a : Inport
  b : Inport  Port=2
  Compare To Zero : simulink/Logic and Bit Operations/Compare To Zero  relop=<=  OutDataTypeStr=boolean
  Multiport Switch2 : MultiPortSwitch  DataPortOrder=Zero-based contiguous  Inputs=2  zeroidx=on
  Subtract18 : Sum  Inputs=+-  OutDataTypeStr=fixdt(1,(w+1)*2+2,f*2)  SaturateOnIntegerOverflow=on
  min : Outport
  wires:
  Compare To Zero/1 -> Multiport Switch2/1
  Multiport Switch2/1 -> min/1
  a/1 -> Subtract18/1, Multiport Switch2/3
  b/1 -> Multiport Switch2/2, Subtract18/2
  Subtract18/1 -> Compare To Zero/1

== matlab function llr/Soft Demodulation 0/symmetric_saturation ==
  data: u input; y output
function y = symmetric_saturation(u)
    if u > 7.75
        y = fi(7.75, 1, 6, 2);
    elseif u < -7.75
        y = fi(-7.75, 1, 6, 2);
    else
        y = fi(u, 1, 6, 2);
    end
